simulink model "TwoEyesModel"  (R2020a)
settings: Solver=FixedStepAuto  StartTime=0.0  StopTime=Tsim  FixedStep=0.1  RelTol=1e-3
values from neighbouring files (symbols this model uses):
  B = 0    [initParamOptimMedianExample.mat]
  H = pOpt(1).Value    [estimateParamsMedian.m]    (also in initParamOptimMedianExample.mat = 6)
  K = pOpt(2).Value    [estimateParamsMedian.m]    (also in initParamOptimMedianExample.mat = 0.6)
  Ka = pOpt(3).Value    [estimateParamsMedian.m]    (also in initParamOptimMedianExample.mat = 1.2)
  Kh = pOpt(4).Value    [estimateParamsMedian.m]    (also in initParamOptimMedianExample.mat = 5.2)
  Kvsm = pOpt(5).Value    [estimateParamsMedian.m]    (also in initParamOptimMedianExample.mat = 0.5)
  Ta = pOpt(6).Value    [estimateParamsMedian.m]    (also in initParamOptimMedianExample.mat = 1000)
  Th = pOpt(7).Value    [estimateParamsMedian.m]    (also in initParamOptimMedianExample.mat = 10)
  Tvsm = pOpt(8).Value    [estimateParamsMedian.m]    (also in initParamOptimMedianExample.mat = 30)
undefined symbols (not defined in the file or in its folder): Ngain1, Ngain2, Tgain1, Tgain2
settings Model: OrderedModelArguments=off  Creator=mmoham53  LastModifiedBy=mmoham53

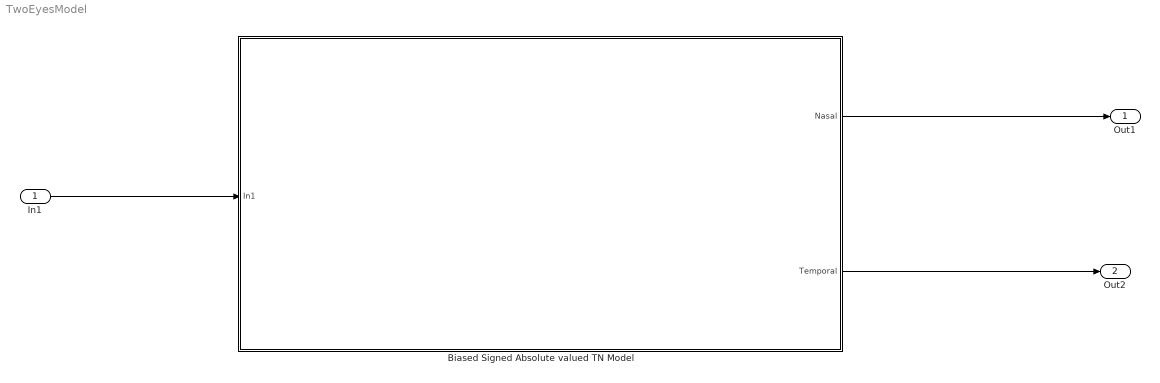
== system TwoEyesModel ==
  In1 : Inport
  Biased Signed Absolute valued TN Model : Subsystem  mask{K=K, Ka=Ka, H=H, Kh=Kh, Ta=Ta, Tvsm=Tvsm, Th=Th, Ngain1=Ngain1, Tgain1=Tgain1, Ngain2=Ngain2, Tgain2=Tgain2, B=B}
      mask prompts: K "Oculomotor gain"; Ka "Adaptation gain"; H "Habitation feedfroward gain"; Kh "Habituation gain"; Ta "Adaptation time constant"; Tvsm "Velocity storage time constant"; Th "Habitation time-constant"; Ngain1 "Nasal gain 1"; Tgain1 "Temporal gain 1"; Ngain2 "Nasal gain 2"; Tgain2 "Temporal gain2"; B "Bias"
  Out1 : Outport
  Out2 : Outport  Port=2
  wires:
  In1/1 -> Biased Signed Absolute valued TN Model/1(In1)
  Biased Signed Absolute valued TN Model/1(Nasal) -> Out1/1
  Biased Signed Absolute valued TN Model/2(Temporal) -> Out2/1

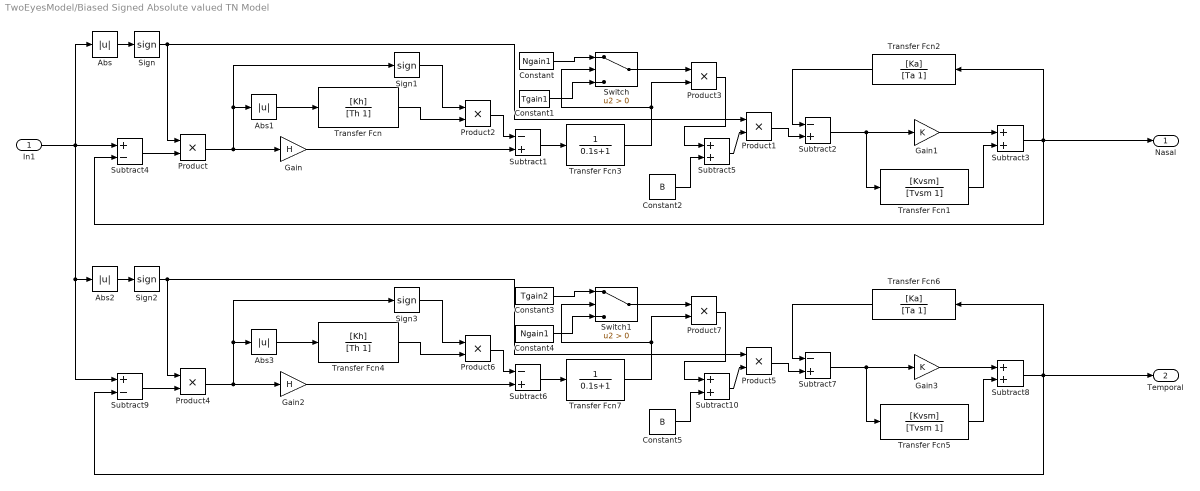
== system TwoEyesModel/Biased Signed Absolute valued TN Model ==
  In1 : Inport
  Abs{,1..3} (4 alike) : Abs
  Constant : Constant  Value=Ngain1
  Constant1 : Constant  Value=Tgain1
  Constant2 : Constant  Value=B
  Constant3 : Constant  Value=Tgain2
  Constant4 : Constant  Value=Ngain1
  Constant5 : Constant  Value=B
  Gain : Gain  Gain=H
  Gain1 : Gain  Gain=K
  Gain2 : Gain  Gain=H
  Gain3 : Gain  Gain=K
  Product{,1..7} (8 alike) : Product
  Sign{,1..3} (4 alike) : Signum
  Subtract{1..2,6..7} (4 alike) : Sum  Inputs=-+
  Subtract{3,5,8,10} (4 alike) : Sum
  Subtract4 : Sum  Inputs=+-
  Subtract9 : Sum  Inputs=+-
  Switch : Switch  Criteria=u2 > Threshold
  Switch1 : Switch  Criteria=u2 > Threshold
  Transfer Fcn : TransferFcn  Numerator=[Kh]  Denominator=[Th 1]
  Transfer Fcn1 : TransferFcn  Numerator=[Kvsm]  Denominator=[Tvsm 1]
  Transfer Fcn2 : TransferFcn  Numerator=[Ka]  Denominator=[Ta 1]
  Transfer Fcn3 : TransferFcn  Denominator=[0.1 1]
  Transfer Fcn4 : TransferFcn  Numerator=[Kh]  Denominator=[Th 1]
  Transfer Fcn5 : TransferFcn  Numerator=[Kvsm]  Denominator=[Tvsm 1]
  Transfer Fcn6 : TransferFcn  Numerator=[Ka]  Denominator=[Ta 1]
  Transfer Fcn7 : TransferFcn  Denominator=[0.1 1]
  Nasal : Outport
  Temporal : Outport  Port=2
  wires:
  Constant2/1 -> Subtract5/2
  Subtract3/1 -> Nasal/1, Subtract4/2, Transfer Fcn2/1
  Abs1/1 -> Transfer Fcn/1
  Subtract4/1 -> Product/2
  Sign1/1 -> Product2/1
  Constant1/1 -> Switch/3
  Product2/1 -> Subtract1/1
  Gain/1 -> Subtract1/2
  Sign/1 -> Product/1, Product1/1
  Transfer Fcn/1 -> Product2/2
  Subtract1/1 -> Transfer Fcn3/1
  Transfer Fcn3/1 -> Product3/2, Switch/2
  Subtract2/1 -> Transfer Fcn1/1, Gain1/1
  Product/1 -> Sign1/1, Abs1/1, Gain/1
  Constant/1 -> Switch/1
  Gain1/1 -> Subtract3/1
  Abs/1 -> Sign/1
  Transfer Fcn1/1 -> Subtract3/2
  Product1/1 -> Subtract2/2
  Transfer Fcn2/1 -> Subtract2/1
  Subtract5/1 -> Product1/2
  Switch/1 -> Product3/1
  Product3/1 -> Subtract5/1
  Switch1/1 -> Product7/1
  Gain2/1 -> Subtract6/2
  Gain3/1 -> Subtract8/1
  Sign3/1 -> Product6/1
  Transfer Fcn6/1 -> Subtract7/1
  Product5/1 -> Subtract7/2
  Subtract7/1 -> Transfer Fcn5/1, Gain3/1
  Constant5/1 -> Subtract10/2
  Abs2/1 -> Sign2/1
  Transfer Fcn4/1 -> Product6/2
  Constant3/1 -> Switch1/1
  Abs3/1 -> Transfer Fcn4/1
  Subtract10/1 -> Product5/2
  Transfer Fcn5/1 -> Subtract8/2
  Transfer Fcn7/1 -> Product7/2, Switch1/2
  Constant4/1 -> Switch1/3
  Product4/1 -> Sign3/1, Abs3/1, Gain2/1
  Subtract6/1 -> Transfer Fcn7/1
  Sign2/1 -> Product4/1, Product5/1
  Subtract9/1 -> Product4/2
  Subtract8/1 -> Temporal/1, Subtract9/2, Transfer Fcn6/1
  Product7/1 -> Subtract10/1
  Product6/1 -> Subtract6/1
  In1/1 -> Subtract9/1, Abs2/1, Subtract4/1, Abs/1
